simulink model "RELOrigin"  (R2022a)
settings: configuration reference "ChildModel" (kept outside this file)
libraries: simulink x4
(part 1 of 2)
settings Model: Creator=Seong Thai  LastModifiedBy=PC
settings ConfigSetRef: SourceName=ChildModel  SourceLocation=Base Workspace

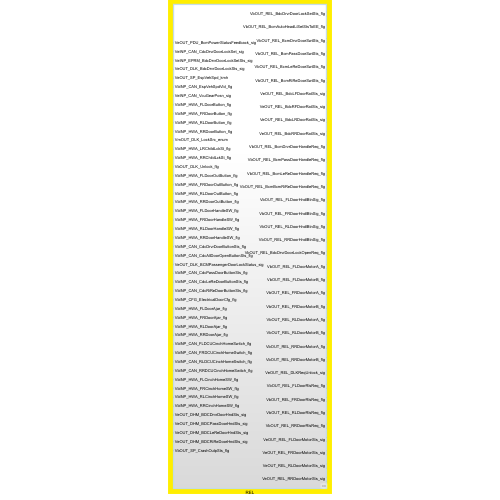
[thumbnail: Simulink's stored preview of the top-level diagram]
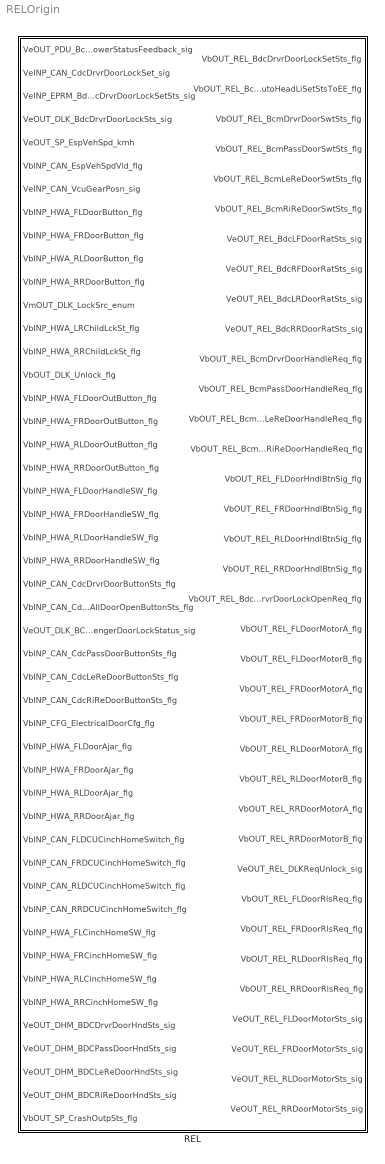
== system RELOrigin ==
  REL : Subsystem

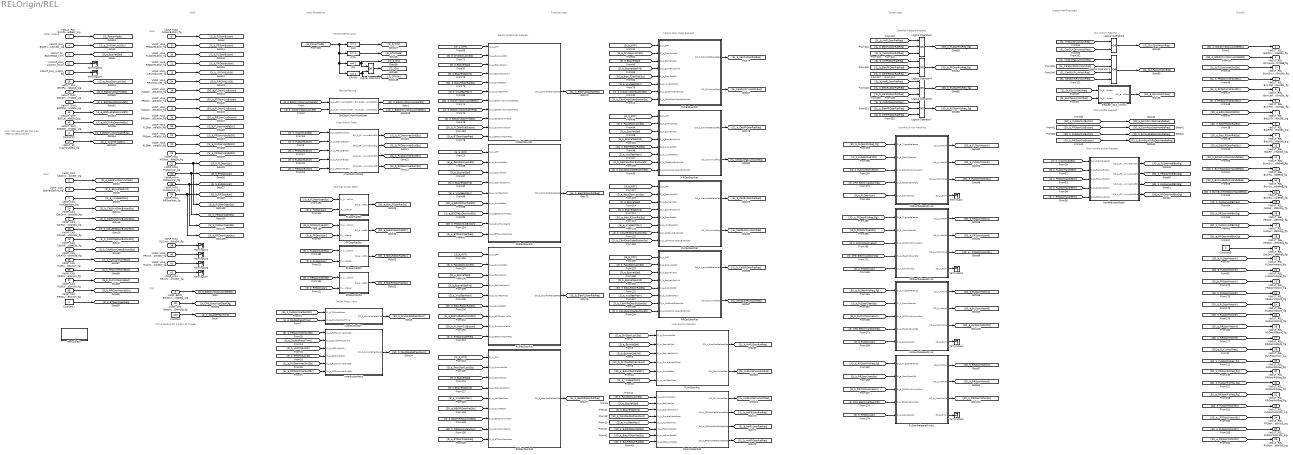
== system RELOrigin/REL ==
  note: Only NFC and BT got this Req
      | //830 no need present
  note: //Time Pending for 2 Press as Trigger
  note: CAN
  note: HWA
  note: Function Logic
  note: Input
  note: Output
  note: Input-Presetting
  note: Other Module
  note: CFG
  note: PowerMode Divation
  note: Inner Button Request
  note: Setting Passing
  note: Inner Button State
  note: Double Press Valid
  note: DoorRat Actual State
  note: Driver Logic
  note: Output Handling Logic
  note: DLK Unlock Request
  note: Door Handle Request
  note: Door Handle Button Request
  note: Electro Slide Open Request
  note: Central Door Open Request
  note: DoorRat Release Request
  note: DoorRat Driver Handling
  VeOUT_PDU_BcmPowerStatusFeedback_sig : Inport
  VeINP_CAN_CdcDrvrDoorLockSet_sig : Inport  Port=2
  VeINP_EPRM_BdcDrvrDoorLockSetSts_sig : Inport  Port=3
  VeOUT_DLK_BdcDrvrDoorLockSts_sig : Inport  Port=4
  VeOUT_SP_EspVehSpd_kmh : Inport  Port=5
  VbINP_CAN_EspVehSpdVld_flg : Inport  Port=6
  VeINP_CAN_VcuGearPosn_sig : Inport  Port=7
  VbINP_HWA_FLDoorButton_flg : Inport  Port=8
  VbINP_HWA_FRDoorButton_flg : Inport  Port=9
  VbINP_HWA_RLDoorButton_flg : Inport  Port=10
  VbINP_HWA_RRDoorButton_flg : Inport  Port=11
  VmOUT_DLK_LockSrc_enum : Inport  Port=12
  VbINP_HWA_LRChildLckSt_flg : Inport  Port=13
  VbINP_HWA_RRChildLckSt_flg : Inport  Port=14
  VbOUT_DLK_Unlock_flg : Inport  Port=15
  VbINP_HWA_FLDoorOutButton_flg : Inport  Port=16
  VbINP_HWA_FRDoorOutButton_flg : Inport  Port=17
  VbINP_HWA_RLDoorOutButton_flg : Inport  Port=18
  VbINP_HWA_RRDoorOutButton_flg : Inport  Port=19
  VbINP_HWA_FLDoorHandleSW_flg : Inport  Port=20
  VbINP_HWA_FRDoorHandleSW_flg : Inport  Port=21
  VbINP_HWA_RLDoorHandleSW_flg : Inport  Port=22
  VbINP_HWA_RRDoorHandleSW_flg : Inport  Port=23
  VbINP_CAN_CdcDrvrDoorButtonSts_flg : Inport  Port=24
  VbINP_CAN_CdcAllDoorOpenButtonSts_flg : Inport  Port=25
  VeOUT_DLK_BCMPassengerDoorLockStatus_sig : Inport  Port=26
  VbINP_CAN_CdcPassDoorButtonSts_flg : Inport  Port=27
  VbINP_CAN_CdcLeReDoorButtonSts_flg : Inport  Port=28
  VbINP_CAN_CdcRiReDoorButtonSts_flg : Inport  Port=29
  VbINP_CFG_ElectricalDoorCfg_flg : Inport  Port=30
  VbINP_HWA_FLDoorAjar_flg : Inport  Port=31
  VbINP_HWA_FRDoorAjar_flg : Inport  Port=32
  VbINP_HWA_RLDoorAjar_flg : Inport  Port=33
  VbINP_HWA_RRDoorAjar_flg : Inport  Port=34
  VbINP_CAN_FLDCUCinchHomeSwitch_flg : Inport  Port=35
  VbINP_CAN_FRDCUCinchHomeSwitch_flg : Inport  Port=36
  VbINP_CAN_RLDCUCinchHomeSwitch_flg : Inport  Port=37
  VbINP_CAN_RRDCUCinchHomeSwitch_flg : Inport  Port=38
  VbINP_HWA_FLCinchHomeSW_flg : Inport  Port=39
  VbINP_HWA_FRCinchHomeSW_flg : Inport  Port=40
  VbINP_HWA_RLCinchHomeSW_flg : Inport  Port=41
  VbINP_HWA_RRCinchHomeSW_flg : Inport  Port=42
  VeOUT_DHM_BDCDrvrDoorHndSts_sig : Inport  Port=43
  VeOUT_DHM_BDCPassDoorHndSts_sig : Inport  Port=44
  VeOUT_DHM_BDCLeReDoorHndSts_sig : Inport  Port=45
  VeOUT_DHM_BDCRiReDoorHndSts_sig : Inport  Port=46
  VbOUT_SP_CrashOutpSts_flg : Inport  Port=47
  CRANK : simulink/Logic and Bit Operations/Compare To Constant  relop===  const=3  OutDataTypeStr=boolean
  Constant : Constant  Value=200
  Constant1 : Constant  Value=0  OutDataTypeStr=uint8
  Constant2 : Constant  Value=0  OutDataTypeStr=boolean
  Constant3 : Constant  Value=0  OutDataTypeStr=boolean
  DrvDoorUnlockAutoOpen : Stateflow chart  TreatAsAtomicUnit=on
  FLCenDoorRat : Stateflow chart  TreatAsAtomicUnit=on
  FLDoorRatSts : Truth Table  TreatAsAtomicUnit=on
  FLDoorReleaseDriver : Stateflow chart  TreatAsAtomicUnit=on
  FLElecDoorRat : Stateflow chart  TreatAsAtomicUnit=on
  FLInnDoorRat : Stateflow chart  TreatAsAtomicUnit=on
  FRCenDoorRat : Stateflow chart  TreatAsAtomicUnit=on
  FRDoorRatSts : Truth Table  TreatAsAtomicUnit=on
  FRDoorReleaseDriver : Stateflow chart  TreatAsAtomicUnit=on
  FRElecDoorRat : Stateflow chart  TreatAsAtomicUnit=on
      settings: PortSchema="{\"entries\":[{\"content\":{\"sides\":[{\"content\":{\"connectorIds\":[\"In1\",\"In2\",\"In3\",\"In4\",\"In6\",\"In5\",\"In7\",\"In8\",\"In9\"]},\"type\":\"ConnectorPlacement.EquallySpacedRectSide\",\"uuid\":\"212e0ac4-578e-4dce-a8b0-108228799b81\"},{\"content\":{\"connectorIds\":[\"Out1\"],\"side\":\"RIGHT\"},\"type\":\"ConnectorPlacement.EquallySpacedRectSide\",\"uuid\":\"8fdf6a0d-489b-40c2-bb8d-375db94844e2\"},{\"content\":{\"connectorIds\":[],\"side\":\"TOP\"},\"type\":\"ConnectorPlacement.EquallySpacedRectSide\",\"uuid\":\"a80be6d9-6bfe-49a2-ae65-45f3c0c1dec5\"}]},\"type\":\"ConnectorPlacement.EquallySpacedConnector\",\"uuid\":\"25043fbd-39b7-455b-b12b-f3efbe7587dc\"}],\"packageUris\":[\"http://schema.mathworks.com/mf0/Connector/R2020b\"],\"version\":\"1.0\"}"
  HandleButtonState : Stateflow chart  TreatAsAtomicUnit=on
  InnerButtonDrv : Stateflow chart  TreatAsAtomicUnit=on
  InnerButtonPass : Stateflow chart  TreatAsAtomicUnit=on
  InnerButtonState : Stateflow chart  TreatAsAtomicUnit=on
  Logical Operator1 : Logic  Operator=OR  Inputs=4  AllPortsSameDT=off  OutDataTypeStr=boolean
  Logical Operator{2,4,6..7} (4 alike) : Logic  Operator=OR  Inputs=3  AllPortsSameDT=off  OutDataTypeStr=boolean
  Logical Operator3 : Logic  Operator=OR  AllPortsSameDT=off  OutDataTypeStr=boolean
  Logical Operator5 : Logic  Operator=OR  AllPortsSameDT=off  OutDataTypeStr=boolean
  "OFF " : simulink/Logic and Bit Operations/Compare To Constant  relop===  const=0  OutDataTypeStr=boolean
  ON : simulink/Logic and Bit Operations/Compare To Constant  relop===  const=2  OutDataTypeStr=boolean
  OTA : simulink/Logic and Bit Operations/Compare To Constant  relop===  const=1  OutDataTypeStr=boolean
  PassInnDoorRat : Stateflow chart  TreatAsAtomicUnit=on
      settings: PortSchema="{\"entries\":[{\"content\":{\"sides\":[{\"content\":{\"connectorIds\":[\"In1\",\"In2\",\"In3\",\"In4\",\"In6\",\"In5\",\"In8\",\"In7\"]},\"type\":\"ConnectorPlacement.EquallySpacedRectSide\",\"uuid\":\"5836de3c-4cf2-45a4-8dc0-e048cbbd381d\"},{\"content\":{\"connectorIds\":[\"Out1\",\"Out2\",\"Out3\",\"Out4\"],\"side\":\"RIGHT\"},\"type\":\"ConnectorPlacement.EquallySpacedRectSide\",\"uuid\":\"b6d6f1b8-f80b-4d0e-a26e-7cda05dade9a\"},{\"content\":{\"connectorIds\":[],\"side\":\"TOP\"},\"type\":\"ConnectorPlacement.EquallySpacedRectSide\",\"uuid\":\"870e6a56-16d5-491b-84d0-76547b1cbcf9\"}]},\"type\":\"ConnectorPlacement.EquallySpacedConnector\",\"uuid\":\"60f0a081-1e33-4aae-8a09-fe9fb7bd0b5c\"}],\"packageUris\":[\"http://schema.mathworks.com/mf0/Connector/R2020b\"],\"version\":\"1.0\"}"
  RLCenDoorRat : Stateflow chart  TreatAsAtomicUnit=on
  RLDoorRatSts : Truth Table  TreatAsAtomicUnit=on
  RLDoorReleaseDriver : Stateflow chart  TreatAsAtomicUnit=on
  RLDoorReleaseDriver1 : Stateflow chart  TreatAsAtomicUnit=on
  RLElecDoorRat : Stateflow chart  TreatAsAtomicUnit=on
      settings: PortSchema="{\"entries\":[{\"content\":{\"sides\":[{\"content\":{\"connectorIds\":[\"In1\",\"In2\",\"In3\",\"In4\",\"In6\",\"In5\",\"In7\",\"In8\",\"In9\"]},\"type\":\"ConnectorPlacement.EquallySpacedRectSide\",\"uuid\":\"212e0ac4-578e-4dce-a8b0-108228799b81\"},{\"content\":{\"connectorIds\":[\"Out1\"],\"side\":\"RIGHT\"},\"type\":\"ConnectorPlacement.EquallySpacedRectSide\",\"uuid\":\"8fdf6a0d-489b-40c2-bb8d-375db94844e2\"},{\"content\":{\"connectorIds\":[],\"side\":\"TOP\"},\"type\":\"ConnectorPlacement.EquallySpacedRectSide\",\"uuid\":\"a80be6d9-6bfe-49a2-ae65-45f3c0c1dec5\"}]},\"type\":\"ConnectorPlacement.EquallySpacedConnector\",\"uuid\":\"25043fbd-39b7-455b-b12b-f3efbe7587dc\"}],\"packageUris\":[\"http://schema.mathworks.com/mf0/Connector/R2020b\"],\"version\":\"1.0\"}"
  RRCenDoorRat : Stateflow chart  TreatAsAtomicUnit=on
  RRDoorRatSts : Truth Table  TreatAsAtomicUnit=on
  RRElecDoorRat : Stateflow chart  TreatAsAtomicUnit=on
      settings: PortSchema="{\"entries\":[{\"content\":{\"sides\":[{\"content\":{\"connectorIds\":[\"In1\",\"In2\",\"In3\",\"In4\",\"In6\",\"In5\",\"In7\",\"In8\",\"In9\"]},\"type\":\"ConnectorPlacement.EquallySpacedRectSide\",\"uuid\":\"212e0ac4-578e-4dce-a8b0-108228799b81\"},{\"content\":{\"connectorIds\":[\"Out1\"],\"side\":\"RIGHT\"},\"type\":\"ConnectorPlacement.EquallySpacedRectSide\",\"uuid\":\"8fdf6a0d-489b-40c2-bb8d-375db94844e2\"},{\"content\":{\"connectorIds\":[],\"side\":\"TOP\"},\"type\":\"ConnectorPlacement.EquallySpacedRectSide\",\"uuid\":\"a80be6d9-6bfe-49a2-ae65-45f3c0c1dec5\"}]},\"type\":\"ConnectorPlacement.EquallySpacedConnector\",\"uuid\":\"25043fbd-39b7-455b-b12b-f3efbe7587dc\"}],\"packageUris\":[\"http://schema.mathworks.com/mf0/Connector/R2020b\"],\"version\":\"1.0\"}"
  Recycle Bin : Subsystem
  Request_DLK_Unlock : Stateflow chart  TreatAsAtomicUnit=on
  Terminator{,1..9} (10 alike) : Terminator
  VbOUT_REL_BdcDrvrDoorLockSetSts_flg : Outport
  VbOUT_REL_BcmAutoHeadLiSetStsToEE_flg : Outport  Port=2
  VbOUT_REL_BcmDrvrDoorSwtSts_flg : Outport  Port=3
  VbOUT_REL_BcmPassDoorSwtSts_flg : Outport  Port=4
  VbOUT_REL_BcmLeReDoorSwtSts_flg : Outport  Port=5
  VbOUT_REL_BcmRiReDoorSwtSts_flg : Outport  Port=6
  VeOUT_REL_BdcLFDoorRatSts_sig : Outport  Port=7
  VeOUT_REL_BdcRFDoorRatSts_sig : Outport  Port=8
  VeOUT_REL_BdcLRDoorRatSts_sig : Outport  Port=9
  VeOUT_REL_BdcRRDoorRatSts_sig : Outport  Port=10
  VbOUT_REL_BcmDrvrDoorHandleReq_flg : Outport  Port=11
  VbOUT_REL_BcmPassDoorHandleReq_flg : Outport  Port=12
  VbOUT_REL_BcmLeReDoorHandleReq_flg : Outport  Port=13
  VbOUT_REL_BcmBcmRiReDoorHandleReq_flg : Outport  Port=14
  VbOUT_REL_FLDoorHndlBtnSig_flg : Outport  Port=15
  VbOUT_REL_FRDoorHndlBtnSig_flg : Outport  Port=16
  VbOUT_REL_RLDoorHndlBtnSig_flg : Outport  Port=17
  VbOUT_REL_RRDoorHndlBtnSig_flg : Outport  Port=18
  VbOUT_REL_BdcDrvrDoorLockOpenReq_flg : Outport  Port=19
  VbOUT_REL_FLDoorMotorA_flg : Outport  Port=20
  VbOUT_REL_FLDoorMotorB_flg : Outport  Port=21
  VbOUT_REL_FRDoorMotorA_flg : Outport  Port=22
  VbOUT_REL_FRDoorMotorB_flg : Outport  Port=23
  VbOUT_REL_RLDoorMotorA_flg : Outport  Port=24
  VbOUT_REL_RLDoorMotorB_flg : Outport  Port=25
  VbOUT_REL_RRDoorMotorA_flg : Outport  Port=26
  VbOUT_REL_RRDoorMotorB_flg : Outport  Port=27
  VeOUT_REL_DLKReqUnlock_sig : Outport  Port=28
  VbOUT_REL_FLDoorRlsReq_flg : Outport  Port=29
  VbOUT_REL_FRDoorRlsReq_flg : Outport  Port=30
  VbOUT_REL_RLDoorRlsReq_flg : Outport  Port=31
  VbOUT_REL_RRDoorRlsReq_flg : Outport  Port=32
  VeOUT_REL_FLDoorMotorSts_sig : Outport  Port=33
  VeOUT_REL_FRDoorMotorSts_sig : Outport  Port=34
  VeOUT_REL_RLDoorMotorSts_sig : Outport  Port=35
  VeOUT_REL_RRDoorMotorSts_sig : Outport  Port=36
  wires:
  "OFF "/1 -> [SI_b_OFF]
  [SI_PowerMode] -> "OFF "/1, CRANK/1, ON/1, OTA/1
  ON/1 -> [SI_b_ON], Logical Operator3/1
  CRANK/1 -> [SI_CRANK], Logical Operator3/2
  Logical Operator3/1 -> [SI_IGN]
  OTA/1 -> [SI_OTAMode]
  VeINP_EPRM_BdcDrvrDoorLockSetSts_sig/1 -> [SI_e_BdcDrvrDoorLockSetSts]
  [SO_b_BdcDrvrDoorLockSetSts] -> VbOUT_REL_BdcDrvrDoorLockSetSts_flg/1
  [SI_e_BdcDrvrDoorLockSetSts] -> DrvDoorUnlockAutoOpen/1(SI_e_BdcDrvrDoorLockSetSts)
  DrvDoorUnlockAutoOpen/1(SO_b_BdcDrvrDoorLockSetSts) -> [SO_b_BdcDrvrDoorLockSetSts]
  VeINP_CAN_CdcDrvrDoorLockSet_sig/1 -> [SI_e_CdcDrvrDoorLockSet]
  [SI_e_CdcDrvrDoorLockSet] -> DrvDoorUnlockAutoOpen/2(SI_e_CdcDrvrDoorLockSet)
  VeOUT_DLK_BdcDrvrDoorLockSts_sig/1 -> [SI_e_DrvDoorLockSts]
  VeOUT_SP_EspVehSpd_kmh/1 -> [SI_e_EspVehSpd]
  VbINP_CAN_EspVehSpdVld_flg/1 -> [SI_b_EspVehSpdVld]
  VbINP_HWA_FLDoorButton_flg/1 -> [SI_b_FLDoorButton]
  [SI_e_DoublePressTime] -> InnerButtonDrv/2(SI_e_DoublePressTime)
  Constant/1 -> [SI_e_DoublePressTime]
  InnerButtonDrv/1(SO_b_DoublePressSucc) -> [SO_b_DrvDoublePressSucc]
  [SI_e_EspVehSpd] -> FLInnDoorRat/2(SI_e_EspVehSpd)
  [SI_b_EspVehSpdVld] -> FLInnDoorRat/3(SI_b_EspVehSpdVld)
  [SO_b_DrvDoublePressSucc] -> FLInnDoorRat/4(SI_b_DoublePressSucc)
  VeINP_CAN_VcuGearPosn_sig/1 -> [SI_e_VcuGearPosn]
  [SI_e_VcuGearPosn] -> FLInnDoorRat/6(SI_e_VcuGearPosn)
  VeOUT_DLK_BCMPassengerDoorLockStatus_sig/1 -> [SI_e_PassDoorLockSts]
  [SI_e_DrvDoorLockSts] -> FLInnDoorRat/1(SI_e_DoorLockSts)
  [SI_e_EspVehSpd] -> PassInnDoorRat/2(SI_e_EspVehSpd)
  [SI_b_EspVehSpdVld] -> PassInnDoorRat/3(SI_b_EspVehSpdVld)
  [SI_e_PassDoorLockSts] -> PassInnDoorRat/1(SI_e_DoorLockSts)
  [SI_e_VcuGearPosn] -> PassInnDoorRat/6(SI_e_VcuGearPosn)
  [SI_e_DoublePressTime] -> InnerButtonPass/2(SI_e_DoublePressTime)
  VbINP_HWA_FRDoorButton_flg/1 -> [SI_b_FRDoorButton]
  VbINP_HWA_LRChildLckSt_flg/1 -> [SI_b_LRChildLckSt]
  VbINP_HWA_RRChildLckSt_flg/1 -> [SI_b_RRChildLckSt]
  [SI_b_LRChildLckSt] -> InnerButtonPass/3(SI_b_LRChildLckSt)
  [SI_b_RRChildLckSt] -> InnerButtonPass/4(SI_b_RRChildLckSt)
  VbINP_CAN_CdcDrvrDoorButtonSts_flg/1 -> [SI_b_CdcDrvrDoorButtonSts]
  VbINP_CAN_CdcPassDoorButtonSts_flg/1 -> [SI_b_CdcPassDoorButtonSts]
  VbINP_CAN_CdcLeReDoorButtonSts_flg/1 -> [SI_b_CdcLeReDoorButtonSts]
  VbINP_CAN_CdcRiReDoorButtonSts_flg/1 -> [SI_b_CdcRiReDoorButtonSts]
  VbINP_HWA_RLDoorButton_flg/1 -> [SI_b_RLDoorButton]
  VbINP_HWA_RRDoorButton_flg/1 -> [SI_b_RRDoorButton]
  [SL_b_FLDoorInnerSwtSts] -> InnerButtonDrv/1(SI_b_FLDoorButton)
  [SL_b_FRDoorInnerSwtSts] -> InnerButtonPass/1(SL_b_FRDoorInnerSwtSts)
  [SL_b_RLDoorInnerSwtSts] -> InnerButtonPass/5(SL_b_RLDoorInnerSwtSts)
  [SL_b_RRDoorInnerSwtSts] -> InnerButtonPass/6(SL_b_RRDoorInnerSwtSts)
  InnerButtonPass/1(SO_b_DoublePressSucc) -> [SO_b_PassDoublePressSucc]
  [SO_b_PassDoublePressSucc] -> PassInnDoorRat/4(SI_b_DoublePressSucc)
  VbINP_HWA_FLDoorAjar_flg/1 -> [SI_b_FLDoorOpenSts], [SI_b_FLDoorAjar]
  VbINP_HWA_FRDoorAjar_flg/1 -> [SI_b_FRDoorOpenSts], [SI_b_FRDoorAjar]
  VbINP_HWA_RLDoorAjar_flg/1 -> [SI_b_RLDoorOpenSts], [SI_b_RLDoorAjar]
  VbINP_HWA_RRDoorAjar_flg/1 -> [SI_b_RRDoorOpenSts], [SI_b_RRDoorAjar]
  [SI_b_FLDoorOpenSts] -> FLDoorRatSts/1(SI_b_DoorAjarSwt)
  [SI_b_RRDoorAjar] -> RRDoorRatSts/2(SI_b_DoorSlideAjar)
  [SI_b_RLDoorAjar] -> RLDoorRatSts/2(SI_b_DoorSlideAjar)
  [SI_b_FRDoorAjar] -> FRDoorRatSts/2(SI_b_DoorSlideAjar)
  [SI_b_FLDoorAjar] -> FLDoorRatSts/2(SI_b_DoorSlideAjar)
  [SI_b_FRDoorOpenSts] -> FRDoorRatSts/1(SI_b_DoorAjarSwt)
  [SI_b_RLDoorOpenSts] -> RLDoorRatSts/1(SI_b_DoorAjarSwt)
  [SI_b_RRDoorOpenSts] -> RRDoorRatSts/1(SI_b_DoorAjarSwt)
  [SO_e_BdcLFDoorRatSts] -> VeOUT_REL_BdcLFDoorRatSts_sig/1
  [SO_e_BdcRFDoorRatSts] -> VeOUT_REL_BdcRFDoorRatSts_sig/1
  [SO_e_BdcLRDoorRatSts] -> VeOUT_REL_BdcLRDoorRatSts_sig/1
  [SO_e_BdcRRDoorRatSts] -> VeOUT_REL_BdcRRDoorRatSts_sig/1
  FLDoorRatSts/1(SO_e_DoorRatSts) -> [SO_e_BdcLFDoorRatSts]
  FRDoorRatSts/1(SO_e_DoorRatSts) -> [SO_e_BdcRFDoorRatSts]
  RRDoorRatSts/1(SO_e_DoorRatSts) -> [SO_e_BdcRRDoorRatSts]
  RLDoorRatSts/1(SO_e_DoorRatSts) -> [SO_e_BdcLRDoorRatSts]
  [SO_e_BdcLFDoorRatSts] -> FLInnDoorRat/5(SI_e_DoorRatSts)
  [SO_e_BdcRFDoorRatSts] -> PassInnDoorRat/5(SI_e_FRDoorRatSts)
  [SO_e_BdcLRDoorRatSts] -> PassInnDoorRat/8(SI_e_RLDoorRatSts)
  [SO_e_BdcRRDoorRatSts] -> PassInnDoorRat/7(SI_e_RRDoorRatSts)
  [SL_b_FLDoorInnerSwtSts] -> VbOUT_REL_BcmDrvrDoorSwtSts_flg/1
  [SL_b_FRDoorInnerSwtSts] -> VbOUT_REL_BcmPassDoorSwtSts_flg/1
  [SL_b_RLDoorInnerSwtSts] -> VbOUT_REL_BcmLeReDoorSwtSts_flg/1
  [SL_b_RRDoorInnerSwtSts] -> VbOUT_REL_BcmRiReDoorSwtSts_flg/1
  FLInnDoorRat/2(SO_DLKUnlockReq) -> [SL_InnDLKDrvUnlockReq]
  PassInnDoorRat/1(SO_DLKUnlockReq) -> [SL_InnDLKPassUnlockReq]
  [SL_DLKDrvUnlockReq] -> Request_DLK_Unlock/1(SL_DLKDrvUnlockReq)
  [SL_DLKPassUnlockReq] -> Request_DLK_Unlock/2(SL_DLKPassUnlockReq)
  Request_DLK_Unlock/1(SO_e_DLKUnlockReq) -> [SO_e_DLKUnlockReq]
  [SO_e_DLKUnlockReq] -> VeOUT_REL_DLKReqUnlock_sig/1
  VbINP_HWA_FLDoorHandleSW_flg/1 -> [SI_b_FLDoorHandleSW]
  VbINP_HWA_FRDoorHandleSW_flg/1 -> [SI_b_FRDoorHandleSW]
  VbINP_HWA_RLDoorHandleSW_flg/1 -> [SI_b_RLDoorHandleSW]
  VbINP_HWA_RRDoorHandleSW_flg/1 -> [SI_b_RRDoorHandleSW]
  [SO_b_BcmDrvrDoorHandleReq] -> VbOUT_REL_BcmDrvrDoorHandleReq_flg/1
  [SO_b_BcmPassDoorHandleReq] -> VbOUT_REL_BcmPassDoorHandleReq_flg/1
  [SO_b_BcmLeReDoorHandleReq] -> VbOUT_REL_BcmLeReDoorHandleReq_flg/1
  [SO_b_BcmBcmRiReDoorHandleReq] -> VbOUT_REL_BcmBcmRiReDoorHandleReq_flg/1
  VbINP_HWA_FLDoorOutButton_flg/1 -> [SO_b_FLDoorOutButton]
  VbINP_HWA_FRDoorOutButton_flg/1 -> [SO_b_FRDoorOutButton]
  VbINP_HWA_RLDoorOutButton_flg/1 -> [SO_b_RLDoorOutButton]
  VbINP_HWA_RRDoorOutButton_flg/1 -> [SO_b_RRDoorOutButton]
  [SO_b_FLDoorHndlBtnSig] -> VbOUT_REL_FLDoorHndlBtnSig_flg/1
  [SO_b_FRDoorHndlBtnSig] -> VbOUT_REL_FRDoorHndlBtnSig_flg/1
  [SO_b_RLDoorHndlBtnSig] -> VbOUT_REL_RLDoorHndlBtnSig_flg/1
  [SO_b_RRDoorHndlBtnSig] -> VbOUT_REL_RRDoorHndlBtnSig_flg/1
  VeOUT_PDU_BcmPowerStatusFeedback_sig/1 -> [SI_PowerMode]
  [SI_e_DrvDoorLockSts] -> FLElecDoorRat/2(SI_e_DoorLockSts)
  [SI_e_EspVehSpd] -> FLElecDoorRat/3(SI_e_EspVehSpd)
  [SI_b_EspVehSpdVld] -> FLElecDoorRat/4(SI_b_EspVehSpdVld)
  [SO_e_BdcLFDoorRatSts] -> FLElecDoorRat/5(SI_e_DoorRatSts)
  [SI_e_VcuGearPosn] -> FLElecDoorRat/6(SI_e_VcuGearPosn)
  [SI_b_OFF] -> FLElecDoorRat/1(SI_b_OFF)
  [SO_b_BdcDrvrDoorLockSetSts] -> FLElecDoorRat/7(SI_b_BdcDrvrDoorLockSetSts)
  Constant2/1 -> [SI_b_BDCDrvrDoorOpenReq]
  [SI_b_BDCDrvrDoorOpenReq] -> FLElecDoorRat/8(SI_b_BDCDrvrDoorOpenReq)
  VeOUT_DHM_BDCDrvrDoorHndSts_sig/1 -> [SI_e_BDCDrvDoorHndSts]
  [SI_e_BDCDrvDoorHndSts] -> FLElecDoorRat/9(SI_e_BDCDoorHndSts)
  [SO_b_FLDoorOutButton] -> FLElecDoorRat/10(SI_b_DoorHandleSW)
  [SI_e_BTDoorOpenReq] -> FLElecDoorRat/11(SI_e_BTDoorOpenReq)
  Constant1/1 -> [SI_e_BTDoorOpenReq]
  FLCenDoorRat/2(SO_DLKUnlockReq) -> [SL_CenDLKDrvUnlockReq]
  [SO_e_BdcLFDoorRatSts] -> FLCenDoorRat/5(SI_e_DoorRatSts)
  [SI_e_DrvDoorLockSts] -> FLCenDoorRat/2(SI_e_DoorLockSts)
  [SI_e_VcuGearPosn] -> FLCenDoorRat/6(SI_e_VcuGearPosn)
  [SI_b_EspVehSpdVld] -> FLCenDoorRat/4(SI_b_EspVehSpdVld)
  [SI_e_EspVehSpd] -> FLCenDoorRat/3(SI_e_EspVehSpd)
  Logical Operator5/1 -> [SL_DLKDrvUnlockReq]
  [SL_InnDLKDrvUnlockReq] -> Logical Operator5/1
  [SL_CenDLKDrvUnlockReq] -> Logical Operator5/2
  VbINP_CAN_CdcAllDoorOpenButtonSts_flg/1 -> [SI_b_Cdc4DoorOpenButtonSts]
  [SI_b_CdcDrvrDoorButtonSts] -> FLCenDoorRat/7(SI_b_CdcDoorButtonSts)
  [SI_b_Cdc4DoorOpenButtonSts] -> FLCenDoorRat/8(SI_b_Cdc4DoorOpenButtonSts)
  [SI_b_OFF] -> FLCenDoorRat/1(SI_b_OFF)
  [SI_b_OFF] -> FRElecDoorRat/1(SI_b_OFF)
  [SI_e_VcuGearPosn] -> FRElecDoorRat/6(SI_e_VcuGearPosn)
  [SI_b_EspVehSpdVld] -> FRElecDoorRat/4(SI_b_EspVehSpdVld)
  [SI_e_EspVehSpd] -> FRElecDoorRat/3(SI_e_EspVehSpd)
  [SI_e_PassDoorLockSts] -> FRElecDoorRat/2(SI_e_DoorLockSts)
  [SO_e_BdcRFDoorRatSts] -> FRElecDoorRat/5(SI_e_DoorRatSts)
  [SI_e_BTDoorOpenReq] -> FRElecDoorRat/9(SI_e_BTDoorOpenReq)
  [SO_b_FRDoorOutButton] -> FRElecDoorRat/8(SI_b_DoorHandleSW)
  VeOUT_DHM_BDCPassDoorHndSts_sig/1 -> [SI_e_BDCPassDoorHndSts]
  [SI_e_BDCPassDoorHndSts] -> FRElecDoorRat/7(SI_e_BDCDoorHndSts)
  [SI_b_OFF] -> FRCenDoorRat/1(SI_b_OFF)
  [SI_b_Cdc4DoorOpenButtonSts] -> FRCenDoorRat/8(SI_b_Cdc4DoorOpenButtonSts)
  [SI_b_CdcPassDoorButtonSts] -> FRCenDoorRat/7(SI_b_CdcDoorButtonSts)
  [SI_e_EspVehSpd] -> FRCenDoorRat/3(SI_e_EspVehSpd)
  [SI_b_EspVehSpdVld] -> FRCenDoorRat/4(SI_b_EspVehSpdVld)
  [SI_e_VcuGearPosn] -> FRCenDoorRat/6(SI_e_VcuGearPosn)
  [SO_e_BdcRFDoorRatSts] -> FRCenDoorRat/5(SI_e_DoorRatSts)
  FRCenDoorRat/2(SO_DLKUnlockReq) -> [SL_CenDLKPassUnlockReq]
  Logical Operator1/1 -> [SL_DLKPassUnlockReq]
  [SL_InnDLKPassUnlockReq] -> Logical Operator1/1
  [SL_CenDLKPassUnlockReq] -> Logical Operator1/2
  [SI_e_PassDoorLockSts] -> FRCenDoorRat/2(SI_e_DoorLockSts)
  [SI_e_BDCLeReDoorHndSts] -> RLElecDoorRat/7(SI_e_BDCDoorHndSts)
  [SO_b_RLDoorOutButton] -> RLElecDoorRat/8(SI_b_DoorHandleSW)
  [SI_e_BTDoorOpenReq] -> RLElecDoorRat/9(SI_e_BTDoorOpenReq)
  [SO_e_BdcLRDoorRatSts] -> RLElecDoorRat/5(SI_e_DoorRatSts)
  [SI_e_PassDoorLockSts] -> RLElecDoorRat/2(SI_e_DoorLockSts)
  [SI_e_EspVehSpd] -> RLElecDoorRat/3(SI_e_EspVehSpd)
  [SI_b_EspVehSpdVld] -> RLElecDoorRat/4(SI_b_EspVehSpdVld)
  [SI_e_VcuGearPosn] -> RLElecDoorRat/6(SI_e_VcuGearPosn)
  [SI_b_OFF] -> RLElecDoorRat/1(SI_b_OFF)
  VeOUT_DHM_BDCLeReDoorHndSts_sig/1 -> [SI_e_BDCLeReDoorHndSts]
  [SI_e_PassDoorLockSts] -> RLCenDoorRat/2(SI_e_DoorLockSts)
  RLCenDoorRat/2(SO_DLKUnlockReq) -> [SL_CenDLKRLUnlockReq]
  [SO_e_BdcLRDoorRatSts] -> RLCenDoorRat/5(SI_e_DoorRatSts)
  [SI_e_VcuGearPosn] -> RLCenDoorRat/6(SI_e_VcuGearPosn)
  [SI_b_EspVehSpdVld] -> RLCenDoorRat/4(SI_b_EspVehSpdVld)
  [SI_e_EspVehSpd] -> RLCenDoorRat/3(SI_e_EspVehSpd)
  [SI_b_CdcLeReDoorButtonSts] -> RLCenDoorRat/7(SI_b_CdcDoorButtonSts)
  [SI_b_Cdc4DoorOpenButtonSts] -> RLCenDoorRat/8(SI_b_Cdc4DoorOpenButtonSts)
  [SI_b_OFF] -> RLCenDoorRat/1(SI_b_OFF)
  [SL_CenDLKRLUnlockReq] -> Logical Operator1/3
  [SI_b_OFF] -> RRElecDoorRat/1(SI_b_OFF)
  [SI_e_VcuGearPosn] -> RRElecDoorRat/6(SI_e_VcuGearPosn)
  [SI_b_EspVehSpdVld] -> RRElecDoorRat/4(SI_b_EspVehSpdVld)
  [SI_e_EspVehSpd] -> RRElecDoorRat/3(SI_e_EspVehSpd)
  [SI_e_PassDoorLockSts] -> RRElecDoorRat/2(SI_e_DoorLockSts)
  [SI_e_BTDoorOpenReq] -> RRElecDoorRat/9(SI_e_BTDoorOpenReq)
  [SO_e_BdcRRDoorRatSts] -> RRElecDoorRat/5(SI_e_DoorRatSts)
  VeOUT_DHM_BDCRiReDoorHndSts_sig/1 -> [SI_e_BDCRiReDoorHndSts]
  [SI_e_BDCRiReDoorHndSts] -> RRElecDoorRat/7(SI_e_BDCDoorHndSts)
  [SO_b_RRDoorOutButton] -> RRElecDoorRat/8(SI_b_DoorHandleSW)
  [SI_b_OFF] -> RRCenDoorRat/1(SI_b_OFF)
  [SI_b_Cdc4DoorOpenButtonSts] -> RRCenDoorRat/8(SI_b_Cdc4DoorOpenButtonSts)
  [SI_e_EspVehSpd] -> RRCenDoorRat/3(SI_e_EspVehSpd)
  [SI_b_EspVehSpdVld] -> RRCenDoorRat/4(SI_b_EspVehSpdVld)
  [SI_e_VcuGearPosn] -> RRCenDoorRat/6(SI_e_VcuGearPosn)
  [SO_e_BdcLRDoorRatSts] -> RRCenDoorRat/5(SI_e_DoorRatSts)
  RRCenDoorRat/2(SO_DLKUnlockReq) -> [SL_CenDLKRRUnlockReq]
  [SI_e_PassDoorLockSts] -> RRCenDoorRat/2(SI_e_DoorLockSts)
  [SI_b_CdcRiReDoorButtonSts] -> RRCenDoorRat/7(SI_b_CdcDoorButtonSts)
  FLInnDoorRat/1(SO_b_DoorRatRelaseReq) -> [SL_b_InnFLDoorRatReq]
  PassInnDoorRat/2(SO_b_FRDoorRatReleaseReq) -> [SL_b_InnFRDoorRatReq]
  PassInnDoorRat/3(SO_b_RLDoorRatReleaseReq) -> [SL_b_InnRLDoorRatReq]
  PassInnDoorRat/4(SO_b_RRDoorRatReleaseReq) -> [SL_b_InnRRDoorRatReq]
  FLElecDoorRat/1(SO_b_DoorRatRelaseReq) -> [SL_b_ElecFLDoorRatReq]
  FLCenDoorRat/1(SO_b_DoorRatRelaseReq) -> [SL_b_CenFLDoorRatReq]
  FRElecDoorRat/1(SO_b_DoorRatRelaseReq) -> [SL_b_ElecFRDoorRatReq]
  RLElecDoorRat/1(SO_b_DoorRatRelaseReq) -> [SL_b_ElecRLDoorRatReq]
  RRElecDoorRat/1(SO_b_DoorRatRelaseReq) -> [SL_b_ElecRRDoorRatReq]
  FRCenDoorRat/1(SO_b_DoorRatRelaseReq) -> [SL_b_CenFRDoorRatReq]
  RLCenDoorRat/1(SO_b_DoorRatRelaseReq) -> [SL_b_CenRLDoorRatReq]
  RRCenDoorRat/1(SO_b_DoorRatRelaseReq) -> [SL_b_CenRRDoorRatReq]
  [SL_CenDLKRRUnlockReq] -> Logical Operator1/4
  [SO_b_FLDoorOutButton] -> [SO_b_BcmDrvrDoorHandleReq]
  [SO_b_FRDoorOutButton] -> [SO_b_BcmPassDoorHandleReq]
  [SO_b_RLDoorOutButton] -> [SO_b_BcmLeReDoorHandleReq]
  [SO_b_RRDoorOutButton] -> [SO_b_BcmBcmRiReDoorHandleReq]
  Constant3/1 -> VbOUT_REL_BdcDrvrDoorLockOpenReq_flg/1
  [SO_b_FLDoorMotorA] -> VbOUT_REL_FLDoorMotorA_flg/1
  [SO_b_FLDoorMotorB] -> VbOUT_REL_FLDoorMotorB_flg/1
  FLDoorReleaseDriver/2(SO_b_MotorB) -> [SO_b_FLDoorMotorB]
  FLDoorReleaseDriver/1(SO_b_MotorA) -> [SO_b_FLDoorMotorA]
  [SL_b_ElecFLDoorRatReq] -> Logical Operator2/2
  [SL_b_InnFLDoorRatReq] -> Logical Operator2/1
  [SL_b_CenFLDoorRatReq] -> Logical Operator2/3
  [SL_b_InnFRDoorRatReq] -> Logical Operator4/1
  [SL_b_ElecFRDoorRatReq] -> Logical Operator4/2
  [SL_b_CenFRDoorRatReq] -> Logical Operator4/3
  [SL_b_ElecRLDoorRatReq] -> Logical Operator6/2
  [SL_b_InnRLDoorRatReq] -> Logical Operator6/1
  [SL_b_CenRLDoorRatReq] -> Logical Operator6/3
  [SL_b_InnRRDoorRatReq] -> Logical Operator7/1
  [SL_b_ElecRRDoorRatReq] -> Logical Operator7/2
  [SL_b_CenRRDoorRatReq] -> Logical Operator7/3
  [SO_b_FLDoorRlsReq_flg] -> VbOUT_REL_FLDoorRlsReq_flg/1
  [SO_b_FRDoorRlsReq_flg] -> VbOUT_REL_FRDoorRlsReq_flg/1
  [SO_b_RLDoorRlsReq_flg] -> VbOUT_REL_RLDoorRlsReq_flg/1
  [SO_b_RRDoorRlsReq_flg] -> VbOUT_REL_RRDoorRlsReq_flg/1
  Logical Operator2/1 -> [SO_b_FLDoorRlsReq_flg]
  Logical Operator7/1 -> [SO_b_RRDoorRlsReq_flg]
  Logical Operator6/1 -> [SO_b_RLDoorRlsReq_flg]
  Logical Operator4/1 -> [SO_b_FRDoorRlsReq_flg]
  [SO_b_FLDoorRlsReq_flg] -> FLDoorReleaseDriver/1(SI_b_TriggerRelease)
  [SI_b_FLDoorAjar] -> FLDoorReleaseDriver/5(SI_b_DoorAjarSts)
  VbINP_CAN_FLDCUCinchHomeSwitch_flg/1 -> [SI_b_FLCinchHomeSwt]
  VbINP_CAN_FRDCUCinchHomeSwitch_flg/1 -> [SI_b_FRCinchHomeSwt]
  VbINP_CAN_RLDCUCinchHomeSwitch_flg/1 -> [SI_b_RLCinchHomeSwt]
  VbINP_CAN_RRDCUCinchHomeSwitch_flg/1 -> [SI_b_RRCinchHomeSwt]
  [SO_b_FRDoorRlsReq_flg] -> FRDoorReleaseDriver/1(SI_b_TriggerRelease)
  [SO_b_RLDoorRlsReq_flg] -> RLDoorReleaseDriver/1(SI_b_TriggerRelease)
  [SO_b_RRDoorRlsReq_flg] -> RLDoorReleaseDriver1/1(SI_b_TriggerRelease)
  [SI_b_FRDoorAjar] -> FRDoorReleaseDriver/5(SI_b_DoorAjarSts)
  [SI_b_RRDoorAjar] -> RLDoorReleaseDriver1/5(SI_b_DoorAjarSts)
  [SI_b_FLCinchHomeSwt] -> FLDoorReleaseDriver/3(SI_b_DCUCinchHomeSwt)
  [SI_b_FRCinchHomeSwt] -> FRDoorReleaseDriver/3(SI_b_DCUCinchHomeSwt)
  [SI_b_RLCinchHomeSwt] -> RLDoorReleaseDriver/3(SI_b_DCUCinchHomeSwt)
  [SI_b_RRCinchHomeSwt] -> RLDoorReleaseDriver1/3(SI_b_DCUCinchHomeSwt)
  VbINP_CFG_ElectricalDoorCfg_flg/1 -> [SI_CFG_ElectricalDoorCfg]
  [SI_CFG_ElectricalDoorCfg] -> FLDoorReleaseDriver/4(SI_b_ElectricDoorCfg)
  [SI_CFG_ElectricalDoorCfg] -> FRDoorReleaseDriver/4(SI_b_ElectricDoorCfg)
  [SI_CFG_ElectricalDoorCfg] -> RLDoorReleaseDriver/4(SI_b_ElectricDoorCfg)
  [SI_CFG_ElectricalDoorCfg] -> RLDoorReleaseDriver1/4(SI_b_ElectricDoorCfg)
  [SO_b_FRDoorMotorB] -> VbOUT_REL_FRDoorMotorB_flg/1
  [SO_b_RLDoorMotorB] -> VbOUT_REL_RLDoorMotorB_flg/1
  [SO_b_RRDoorMotorB] -> VbOUT_REL_RRDoorMotorB_flg/1
  [SO_b_FRDoorMotorA] -> VbOUT_REL_FRDoorMotorA_flg/1
  [SO_b_RLDoorMotorA] -> VbOUT_REL_RLDoorMotorA_flg/1
  [SO_b_RRDoorMotorA] -> VbOUT_REL_RRDoorMotorA_flg/1
  RLDoorReleaseDriver1/1(SO_b_MotorA) -> [SO_b_RRDoorMotorA]
  RLDoorReleaseDriver1/2(SO_b_MotorB) -> [SO_b_RRDoorMotorB]
  RLDoorReleaseDriver/2(SO_b_MotorB) -> [SO_b_RLDoorMotorB]
  RLDoorReleaseDriver/1(SO_b_MotorA) -> [SO_b_RLDoorMotorA]
  FRDoorReleaseDriver/1(SO_b_MotorA) -> [SO_b_FRDoorMotorA]
  FRDoorReleaseDriver/2(SO_b_MotorB) -> [SO_b_FRDoorMotorB]
  [SO_e_FLDoorMotorSts] -> VeOUT_REL_FLDoorMotorSts_sig/1
  [SO_e__FRDoorMotorSts] -> VeOUT_REL_FRDoorMotorSts_sig/1
  [SO_e_RLDoorMotorSts] -> VeOUT_REL_RLDoorMotorSts_sig/1
  [SO_e_RRDoorMotorSts] -> VeOUT_REL_RRDoorMotorSts_sig/1
  FLDoorReleaseDriver/3(SO_e_MotorMode) -> [SO_e_FLDoorMotorSts]
  FRDoorReleaseDriver/3(SO_e_MotorMode) -> [SO_e__FRDoorMotorSts]
  RLDoorReleaseDriver/3(SO_e_MotorMode) -> [SO_e_RLDoorMotorSts]
  RLDoorReleaseDriver1/3(SO_e_MotorMode) -> [SO_e_RRDoorMotorSts]
  FLDoorReleaseDriver/4(SO_b_Error) -> Terminator/1
  FRDoorReleaseDriver/4(SO_b_Error) -> Terminator1/1
  RLDoorReleaseDriver/4(SO_b_Error) -> Terminator2/1
  RLDoorReleaseDriver1/4(SO_b_Error) -> Terminator3/1
  VbINP_HWA_FLCinchHomeSW_flg/1 -> Terminator4/1
  VbINP_HWA_FRCinchHomeSW_flg/1 -> Terminator5/1
  VbINP_HWA_RLCinchHomeSW_flg/1 -> Terminator6/1
  VbINP_HWA_RRCinchHomeSW_flg/1 -> Terminator7/1
  VmOUT_DLK_LockSrc_enum/1 -> Terminator8/1
  VbOUT_DLK_Unlock_flg/1 -> Terminator9/1
  VbOUT_SP_CrashOutpSts_flg/1 -> [SI_b_CrashOutpSts]
  [SI_b_FLDoorOpenSts] -> FLDoorReleaseDriver/2(SI_b_DoorOpenSts)
  [SI_b_FRDoorOpenSts] -> FRDoorReleaseDriver/2(SI_b_DoorOpenSts)
  [SI_b_RLDoorOpenSts] -> RLDoorReleaseDriver/2(SI_b_DoorOpenSts)
  [SI_b_RLDoorAjar] -> RLDoorReleaseDriver/5(SI_b_DoorAjarSts)
  [SI_b_RRDoorOpenSts] -> RLDoorReleaseDriver1/2(SI_b_DoorOpenSts)
  [SI_b_CrashOutpSts] -> InnerButtonState/1(SI_b_CrashOutpSts)
  [SI_b_FLDoorButton] -> InnerButtonState/2(SI_b_FLDoorButton)
  [SI_b_FRDoorButton] -> InnerButtonState/3(SI_b_FRDoorButton)
  [SI_b_RLDoorButton] -> InnerButtonState/4(SI_b_RLDoorButton)
  [SI_b_RRDoorButton] -> InnerButtonState/5(SI_b_RRDoorButton)
  InnerButtonState/1(SO_b_FLDoorInnerSwtSts) -> [SL_b_FLDoorInnerSwtSts]
  InnerButtonState/2(SO_b_FRDoorInnerSwtSts) -> [SL_b_FRDoorInnerSwtSts]
  InnerButtonState/3(SO_b_RLDoorInnerSwtSts) -> [SL_b_RLDoorInnerSwtSts]
  InnerButtonState/4(SO_b_RRDoorInnerSwtSts) -> [SL_b_RRDoorInnerSwtSts]
  [SI_b_CrashOutpSts] -> HandleButtonState/1(SI_b_CrashOutpSts)
  [SI_b_RRDoorHandleSW] -> HandleButtonState/5(SI_b_RRDoorButton)
  [SI_b_RLDoorHandleSW] -> HandleButtonState/4(SI_b_RLDoorButton)
  [SI_b_FRDoorHandleSW] -> HandleButtonState/3(SI_b_FRDoorButton)
  [SI_b_FLDoorHandleSW] -> HandleButtonState/2(SI_b_FLDoorButton)
  HandleButtonState/3(SO_b_RLDoorInnerSwtSts) -> [SO_b_RLDoorHndlBtnSig]
  HandleButtonState/2(SO_b_FRDoorInnerSwtSts) -> [SO_b_FRDoorHndlBtnSig]
  HandleButtonState/4(SO_b_RRDoorInnerSwtSts) -> [SO_b_RRDoorHndlBtnSig]
  HandleButtonState/1(SO_b_FLDoorInnerSwtSts) -> [SO_b_FLDoorHndlBtnSig]
  DrvDoorUnlockAutoOpen/2(SO_b_E2BdcDrvrDoorLockSetSts) -> [SO_b_E2BdcDrvrDoorLockSetSts]
  [SO_b_E2BdcDrvrDoorLockSetSts] -> VbOUT_REL_BcmAutoHeadLiSetStsToEE_flg/1

== system RELOrigin/REL/Recycle Bin ==

== stateflow chart RELOrigin/REL/InnerButtonState ==
  state Initial
    en:
    SO_b_FLDoorInnerSwtSts=SI_b_FLDoorButton;
    SO_b_FRDoorInnerSwtSts=SI_b_FRDoorButton;
    SO_b_RLDoorInnerSwtSts=SI_b_RLDoorButton;
    SO_b_RRDoorInnerSwtSts=SI_b_RRDoorButton;
    du:
    SO_b_FLDoorInnerSwtSts=SI_b_FLDoorButton;
    SO_b_FRDoorInnerSwtSts=SI_b_FRDoorButton;
    SO_b_RLDoorInnerSwtSts=SI_b_RLDoorButton;
    SO_b_RRDoorInnerSwtSts=SI_b_RRDoorButton;
  state ONCE
    en:
    SO_b_FLDoorInnerSwtSts=0;
    SO_b_FRDoorInnerSwtSts=0;
    SO_b_RLDoorInnerSwtSts=0;
    SO_b_RRDoorInnerSwtSts=0;
  (default) -> Initial
  Initial -> ONCE : [hasChangedTo(SI_b_CrashOutpSts,1)]
  ONCE -> Initial : [after(10000,tick)]
  data: SO_b_FLDoorInnerSwtSts output boolean; SI_b_CrashOutpSts input boolean; SI_b_FLDoorButton input boolean; SI_b_FRDoorButton input boolean; SI_b_RLDoorButton input boolean; SI_b_RRDoorButton input boolean; SO_b_FRDoorInnerSwtSts output boolean; SO_b_RLDoorInnerSwtSts output boolean; SO_b_RRDoorInnerSwtSts output boolean

== stateflow chart RELOrigin/REL/HandleButtonState ==
  state Initial
    en:
    SO_b_FLDoorInnerSwtSts=SI_b_FLDoorButton;
    SO_b_FRDoorInnerSwtSts=SI_b_FRDoorButton;
    SO_b_RLDoorInnerSwtSts=SI_b_RLDoorButton;
    SO_b_RRDoorInnerSwtSts=SI_b_RRDoorButton;
    du:
    SO_b_FLDoorInnerSwtSts=SI_b_FLDoorButton;
    SO_b_FRDoorInnerSwtSts=SI_b_FRDoorButton;
    SO_b_RLDoorInnerSwtSts=SI_b_RLDoorButton;
    SO_b_RRDoorInnerSwtSts=SI_b_RRDoorButton;
  state ONCE
    en:
    SO_b_FLDoorInnerSwtSts=0;
    SO_b_FRDoorInnerSwtSts=0;
    SO_b_RLDoorInnerSwtSts=0;
    SO_b_RRDoorInnerSwtSts=0;
  (default) -> Initial
  Initial -> ONCE : [hasChangedTo(SI_b_CrashOutpSts,1)]
  ONCE -> Initial : [after(10000,tick)]
  data: SO_b_FLDoorInnerSwtSts output boolean; SI_b_CrashOutpSts input boolean; SI_b_FLDoorButton input boolean; SI_b_FRDoorButton input boolean; SI_b_RLDoorButton input boolean; SI_b_RRDoorButton input boolean; SO_b_FRDoorInnerSwtSts output boolean; SO_b_RLDoorInnerSwtSts output boolean; SO_b_RRDoorInnerSwtSts output boolean

== stateflow chart RELOrigin/REL/DrvDoorUnlockAutoOpen ==
  state InitialSet (E2value) [function]
    (default) -> (junction 74)
    (junction 74) -> (junction 76) [order 1] : [SI_e_BdcDrvrDoorLockSetSts==1]
        | {SO_b_BdcDrvrDoorLockSetSts=1;}
    (junction 74) -> (junction 78) [order 2]
    (junction 78) -> (junction 80) : {SO_b_BdcDrvrDoorLockSetSts=0;}
  state Initial
    en:
    InitialSet(SI_e_BdcDrvrDoorLockSetSts);
  state CFG_SETTING
    CFG_SETTING -> (junction 56)
    (junction 56) -> (junction 58) [order 1] : [SI_e_CdcDrvrDoorLockSet==1]
        | {SO_b_BdcDrvrDoorLockSetSts=1;
        | SO_b_E2BdcDrvrDoorLockSetSts=1;}
    (junction 56) -> (junction 60) [order 2]
    (junction 60) -> (junction 62) : {SO_b_BdcDrvrDoorLockSetSts=0;
        | SO_b_E2BdcDrvrDoorLockSetSts=0;}
  (default) -> Initial
  Initial -> CFG_SETTING : [after(100,tick)]
  data: E2value function_input double; SO_b_BdcDrvrDoorLockSetSts output boolean; SI_e_BdcDrvrDoorLockSetSts input uint8; SI_e_CdcDrvrDoorLockSet input uint8; SO_b_E2BdcDrvrDoorLockSetSts output boolean

== stateflow chart RELOrigin/REL/InnerButtonDrv ==
  state Initial
    en:
    SO_b_DoublePressSucc=0;
  state ONCE
  state TWICE
    en:
    SO_b_DoublePressSucc=1;
  (default) -> Initial
  Initial -> ONCE : [hasChangedTo(SI_b_FLDoorButton,1)]
  ONCE -> TWICE [order 1] : [before(SI_e_DoublePressTime,tick)&&...
      | hasChangedTo(SI_b_FLDoorButton,1)]
  ONCE -> Initial [order 2] : [after(SI_e_DoublePressTime,tick)]
  TWICE -> Initial : [after(3,tick)]
  data: SO_b_DoublePressSucc output boolean; SI_b_FLDoorButton input boolean; SI_e_DoublePressTime input uint8

== stateflow chart RELOrigin/REL/PassInnDoorRat ==
  state Initial
    en:
    SO_b_FRDoorRatReleaseReq=0;
    SO_b_RLDoorRatReleaseReq=0;
    SO_b_RRDoorRatReleaseReq=0;
    SO_DLKUnlockReq=0;
  state TRIGGER
    state RELEASE
      (default) -> (junction 88)
      (junction 88) -> (junction 91) [order 1] : [SI_e_FRDoorRatSts!=3]
      (junction 88) -> (junction 90) [order 2]
      (junction 91) -> (junction 94) : {SO_b_FRDoorRatReleaseReq=1;}
      (junction 94) -> (junction 90)
      (junction 90) -> (junction 97)
      (junction 97) -> (junction 100) [order 1] : [SI_e_RLDoorRatSts!=3]
      (junction 97) -> (junction 103) [order 2]
      (junction 100) -> (junction 99) : {SO_b_RLDoorRatReleaseReq=1;}
      (junction 99) -> (junction 103)
      (junction 103) -> (junction 112)
      (junction 112) -> (junction 109) [order 1] : [SI_e_RRDoorRatSts!=3]
      (junction 112) -> (junction 108) [order 2]
      (junction 109) -> (junction 105) : {SO_b_RRDoorRatReleaseReq=1;}
      (junction 105) -> (junction 108)
    state DOOR_LOCK
      state REQ_UNLOCK
        en:
        SO_DLKUnlockReq=1;
      state SUCESS_UNLOCK
      state FAIL_UNLOCK
      (default) -> REQ_UNLOCK
      REQ_UNLOCK -> SUCESS_UNLOCK [order 1] : [SI_e_DoorLockSts==1]
      REQ_UNLOCK -> FAIL_UNLOCK [order 2] : [after(100,tick)&&...
          | SI_e_DoorLockSts==0]
    state DOOR_UNLOCK
    (default) -> DOOR_LOCK [order 1] : [SI_e_DoorLockSts==0]
    DOOR_LOCK -> RELEASE : [SI_e_DoorLockSts==1&&...
        | (SI_e_FRDoorRatSts!=3||...
        | SI_e_RLDoorRatSts!=3||...
        | SI_e_RRDoorRatSts!=3)]
    DOOR_UNLOCK -> RELEASE : [SI_e_DoorLockSts==1&&...
        | (SI_e_FRDoorRatSts!=3||...
        | SI_e_RLDoorRatSts!=3||...
        | SI_e_RRDoorRatSts!=3)]
    (default) -> DOOR_UNLOCK [order 2]
  (default) -> Initial
  Initial -> TRIGGER : [((SI_e_EspVehSpd<=0&&SI_b_EspVehSpdVld==0)||...
      | SI_e_VcuGearPosn==1)&&...
      | hasChangedTo(SI_b_DoublePressSucc,1)]
  TRIGGER -> Initial [order 1] : [hasChangedFrom(SI_e_VcuGearPosn,1)||...
      | (SI_e_EspVehSpd>=5&&SI_b_EspVehSpdVld==0)||...
      | (after(105,tick)&&SI_e_DoorLockSts==0)]
  TRIGGER -> Initial [order 2] : [SI_e_DoorLockSts==1&&...
      | SI_e_FRDoorRatSts==3&&...
      | SI_e_RLDoorRatSts==3&&...
      | SI_e_RRDoorRatSts==3]
  RELEASE -> (junction 82) : [after(5,tick)]
  (junction 82) -> Initial
  data: SI_e_DoorLockSts input uint8; SI_e_EspVehSpd input uint8; SI_b_EspVehSpdVld input boolean; SI_b_DoublePressSucc input boolean; SI_e_FRDoorRatSts input uint8; SO_DLKUnlockReq output boolean; SO_b_FRDoorRatReleaseReq output boolean; SI_e_VcuGearPosn input uint8; SI_e_RRDoorRatSts input uint8; SI_e_RLDoorRatSts input uint8; SO_b_RLDoorRatReleaseReq output boolean; SO_b_RRDoorRatReleaseReq output boolean

== stateflow chart RELOrigin/REL/InnerButtonPass ==
  state MAIN_JUDGE [group]
    state FR_BUTTON [parallel]
      settings: executionOrder=1
      state Initial
        en:
        SL_b_FRDBLPressSucc=0;
      state ONCE
      state TWICE
        en:
        SL_b_FRDBLPressSucc=1;
      (default) -> MAIN_JUDGE.FR_BUTTON.Initial
      MAIN_JUDGE.FR_BUTTON.Initial -> MAIN_JUDGE.FR_BUTTON.ONCE : [hasChangedTo(SL_b_FRDoorInnerSwtSts,1)]
      MAIN_JUDGE.FR_BUTTON.ONCE -> MAIN_JUDGE.FR_BUTTON.TWICE [order 1] : [before(SI_e_DoublePressTime,tick)&&...
          | hasChangedTo(SL_b_FRDoorInnerSwtSts,1)]
      MAIN_JUDGE.FR_BUTTON.ONCE -> MAIN_JUDGE.FR_BUTTON.Initial [order 2] : [after(SI_e_DoublePressTime,tick)]
      MAIN_JUDGE.FR_BUTTON.TWICE -> MAIN_JUDGE.FR_BUTTON.Initial : [after(3,tick)]
    state RL_BUTTON [parallel]
      settings: executionOrder=2
      state Initial
        en:
        SL_b_RLDBLPressSucc=0;
      state ONCE
      state TWICE
        en:
        SL_b_RLDBLPressSucc=1;
      (default) -> MAIN_JUDGE.RL_BUTTON.Initial
      MAIN_JUDGE.RL_BUTTON.Initial -> MAIN_JUDGE.RL_BUTTON.ONCE : [hasChangedTo(SL_b_RLDoorInnerSwtSts,1)&&...
          | SI_b_LRChildLckSt==0]
      MAIN_JUDGE.RL_BUTTON.ONCE -> MAIN_JUDGE.RL_BUTTON.Initial [order 2] : [after(SI_e_DoublePressTime,tick)||...
          | SI_b_LRChildLckSt==0]
      MAIN_JUDGE.RL_BUTTON.ONCE -> MAIN_JUDGE.RL_BUTTON.TWICE [order 1] : [before(SI_e_DoublePressTime,tick)&&...
          | SI_b_LRChildLckSt==0&&...
          | hasChangedTo(SL_b_RLDoorInnerSwtSts,1)]
      MAIN_JUDGE.RL_BUTTON.TWICE -> MAIN_JUDGE.RL_BUTTON.Initial : [after(3,tick)]
    state RR_BUTTON [parallel]
      settings: executionOrder=3
      state Initial
        en:
        SL_b_RRDBLPressSucc=0;
      state ONCE
      state TWICE
        en:
        SL_b_RRDBLPressSucc=1;
      (default) -> MAIN_JUDGE.RR_BUTTON.Initial
      MAIN_JUDGE.RR_BUTTON.Initial -> MAIN_JUDGE.RR_BUTTON.ONCE : [hasChangedTo(SL_b_RRDoorInnerSwtSts,1)&&...
          | SI_b_RRChildLckSt==0]
      MAIN_JUDGE.RR_BUTTON.ONCE -> MAIN_JUDGE.RR_BUTTON.Initial [order 2] : [after(SI_e_DoublePressTime,tick)||...
          | SI_b_RRChildLckSt!=0]
      MAIN_JUDGE.RR_BUTTON.ONCE -> MAIN_JUDGE.RR_BUTTON.TWICE [order 1] : [before(SI_e_DoublePressTime,tick)&&...
          | SI_b_RRChildLckSt==0&&...
          | hasChangedTo(SL_b_RRDoorInnerSwtSts,1)]
      MAIN_JUDGE.RR_BUTTON.TWICE -> MAIN_JUDGE.RR_BUTTON.Initial : [after(3,tick)]
  state OUTPUT_HANDLE [group]
    state OUTPUT [parallel]
      settings: executionOrder=1
      state IDLE
        en:
        SO_b_DoublePressSucc=0;
      state SEND_OUT
        en:
        SO_b_DoublePressSucc=1;
      (default) -> IDLE
      IDLE -> SEND_OUT : [SL_b_FRDBLPressSucc||...
          | SL_b_RLDBLPressSucc||...
          | SL_b_RRDBLPressSucc]
      SEND_OUT -> IDLE : [!SL_b_FRDBLPressSucc&&...
          | !SL_b_RLDBLPressSucc&&...
          | !SL_b_RRDBLPressSucc]
  data: SO_b_DoublePressSucc output boolean; SL_b_FRDoorInnerSwtSts input boolean; SI_e_DoublePressTime input uint8; SI_b_LRChildLckSt input boolean; SI_b_RRChildLckSt input boolean; SL_b_RLDoorInnerSwtSts input boolean; SL_b_RRDoorInnerSwtSts input boolean; SL_b_FRDBLPressSucc local boolean; SL_b_RRDBLPressSucc local boolean; SL_b_RLDBLPressSucc local boolean

== matlab function RELOrigin/REL/FLDoorRatSts ==
  data: SI_b_DoorAjarSwt input boolean; SO_e_DoorRatSts output uint8; SI_b_DoorSlideAjar input boolean
function SO_e_DoorRatSts = fcn(SI_b_DoorAjarSwt, SI_b_DoorSlideAjar)

aVarTruthTableCondition_1 = false;
aVarTruthTableCondition_2 = false;


% Example condition 1

aVarTruthTableCondition_1 = logical(SI_b_DoorAjarSwt==false);

% Example condition 2

aVarTruthTableCondition_2 = logical(SI_b_DoorSlideAjar==false);

if (~aVarTruthTableCondition_1 && ~aVarTruthTableCondition_2)
    aFcnTruthTableAction_2();
elseif (~aVarTruthTableCondition_1 && aVarTruthTableCondition_2)
    aFcnTruthTableAction_3();
elseif (aVarTruthTableCondition_1 && aVarTruthTableCondition_2)
    aFcnTruthTableAction_4();
else % Default
    aFcnTruthTableAction_1();
end

function aFcnTruthTableAction_1()

% Invalid

SO_e_DoorRatSts=0;

function aFcnTruthTableAction_2()

% All Lock

SO_e_DoorRatSts=1;

function aFcnTruthTableAction_3()

% Half Lock

SO_e_DoorRatSts=2;

function aFcnTruthTableAction_4()

% All Unlock

SO_e_DoorRatSts=3;

== matlab function RELOrigin/REL/FRDoorRatSts ==
  data: SI_b_DoorAjarSwt input boolean; SO_e_DoorRatSts output uint8; SI_b_DoorSlideAjar input boolean
function SO_e_DoorRatSts = fcn(SI_b_DoorAjarSwt, SI_b_DoorSlideAjar)

aVarTruthTableCondition_1 = false;
aVarTruthTableCondition_2 = false;


% Example condition 1

aVarTruthTableCondition_1 = logical(SI_b_DoorAjarSwt==false);

% Example condition 2

aVarTruthTableCondition_2 = logical(SI_b_DoorSlideAjar==false);

if (~aVarTruthTableCondition_1 && ~aVarTruthTableCondition_2)
    aFcnTruthTableAction_2();
elseif (~aVarTruthTableCondition_1 && aVarTruthTableCondition_2)
    aFcnTruthTableAction_3();
elseif (aVarTruthTableCondition_1 && aVarTruthTableCondition_2)
    aFcnTruthTableAction_4();
else % Default
    aFcnTruthTableAction_1();
end

function aFcnTruthTableAction_1()

% Invalid

SO_e_DoorRatSts=0;

function aFcnTruthTableAction_2()

% All Lock

SO_e_DoorRatSts=1;

function aFcnTruthTableAction_3()

% Half Lock

SO_e_DoorRatSts=2;

function aFcnTruthTableAction_4()

% All Unlock

SO_e_DoorRatSts=3;

== matlab function RELOrigin/REL/RLDoorRatSts ==
  data: SI_b_DoorAjarSwt input boolean; SO_e_DoorRatSts output uint8; SI_b_DoorSlideAjar input boolean
function SO_e_DoorRatSts = fcn(SI_b_DoorAjarSwt, SI_b_DoorSlideAjar)

aVarTruthTableCondition_1 = false;
aVarTruthTableCondition_2 = false;


% Example condition 1

aVarTruthTableCondition_1 = logical(SI_b_DoorAjarSwt==false);

% Example condition 2

aVarTruthTableCondition_2 = logical(SI_b_DoorSlideAjar==false);

if (~aVarTruthTableCondition_1 && ~aVarTruthTableCondition_2)
    aFcnTruthTableAction_2();
elseif (~aVarTruthTableCondition_1 && aVarTruthTableCondition_2)
    aFcnTruthTableAction_3();
elseif (aVarTruthTableCondition_1 && aVarTruthTableCondition_2)
    aFcnTruthTableAction_4();
else % Default
    aFcnTruthTableAction_1();
end

function aFcnTruthTableAction_1()

% Invalid

SO_e_DoorRatSts=0;

function aFcnTruthTableAction_2()

% All Lock

SO_e_DoorRatSts=1;

function aFcnTruthTableAction_3()

% Half Lock

SO_e_DoorRatSts=2;

function aFcnTruthTableAction_4()

% All Unlock

SO_e_DoorRatSts=3;

== matlab function RELOrigin/REL/RRDoorRatSts ==
  data: SI_b_DoorAjarSwt input boolean; SO_e_DoorRatSts output uint8; SI_b_DoorSlideAjar input boolean
function SO_e_DoorRatSts = fcn(SI_b_DoorAjarSwt, SI_b_DoorSlideAjar)

aVarTruthTableCondition_1 = false;
aVarTruthTableCondition_2 = false;


% Example condition 1

aVarTruthTableCondition_1 = logical(SI_b_DoorAjarSwt==false);

% Example condition 2

aVarTruthTableCondition_2 = logical(SI_b_DoorSlideAjar==false);

if (~aVarTruthTableCondition_1 && ~aVarTruthTableCondition_2)
    aFcnTruthTableAction_2();
elseif (~aVarTruthTableCondition_1 && aVarTruthTableCondition_2)
    aFcnTruthTableAction_3();
elseif (aVarTruthTableCondition_1 && aVarTruthTableCondition_2)
    aFcnTruthTableAction_4();
else % Default
    aFcnTruthTableAction_1();
end

function aFcnTruthTableAction_1()

% Invalid

SO_e_DoorRatSts=0;

function aFcnTruthTableAction_2()

% All Lock

SO_e_DoorRatSts=1;

function aFcnTruthTableAction_3()

% Half Lock

SO_e_DoorRatSts=2;

function aFcnTruthTableAction_4()

% All Unlock

SO_e_DoorRatSts=3;

== stateflow chart RELOrigin/REL/Request_DLK_Unlock ==
  state REQ_SENT
    REQ_SENT -> (junction 56) [order 1]
    (junction 56) -> (junction 58) [order 1] : [SL_DLKDrvUnlockReq==1&&...
        | SL_DLKPassUnlockReq==1]
    (junction 56) -> (junction 60) [order 2]
    (junction 58) -> (junction 91) : {SO_e_DLKUnlockReq=3;}
    (junction 60) -> (junction 62) [order 1] : [SL_DLKDrvUnlockReq==1&&...
        | SL_DLKPassUnlockReq!=1]
    (junction 60) -> (junction 84) [order 2]
    (junction 62) -> (junction 93) : {SO_e_DLKUnlockReq=1;}
    (junction 84) -> (junction 83) [order 1] : [SL_DLKDrvUnlockReq!=1&&...
        | SL_DLKPassUnlockReq==1]
    (junction 84) -> (junction 88) [order 2] : {SO_e_DLKUnlockReq=0;}
    (junction 83) -> (junction 95) : {SO_e_DLKUnlockReq=2;}
  state Initial
    en:
    SO_e_DLKUnlockReq=0;
  (default) -> Initial
  Initial -> REQ_SENT : [hasChangedTo(SL_DLKDrvUnlockReq,1)||...
      | hasChangedTo(SL_DLKPassUnlockReq,1)]
  REQ_SENT -> Initial [order 1] : [SL_DLKDrvUnlockReq==0&&...
      | SL_DLKPassUnlockReq==0]
  data: SO_e_DLKUnlockReq output uint8; SL_DLKDrvUnlockReq input boolean; SL_DLKPassUnlockReq input boolean

== stateflow chart RELOrigin/REL/FLElecDoorRat ==
  state Initial
    en:
    SO_b_DoorRatRelaseReq=0;
  state RELEASE
    en:
    SO_b_DoorRatRelaseReq=1;
  (default) -> Initial
  Initial -> RELEASE : [!SI_b_OFF&&...
      | SI_e_DoorLockSts==1&&...
      | SI_e_DoorRatSts!=3&&...
      | ((SI_e_EspVehSpd<=0&&SI_b_EspVehSpdVld==0)||...
      | SI_e_VcuGearPosn==1)&&...
      | ((SI_b_BdcDrvrDoorLockSetSts==1&&SI_b_BDCDrvrDoorOpenReq)||...
      | (SI_e_BDCDoorHndSts==1&&hasChangedTo(SI_b_DoorHandleSW,1))||...
      | (SI_e_VcuGearPosn==1&&hasChangedTo(SI_e_BTDoorOpenReq,1))||...
      | (SI_e_VcuGearPosn==1&&hasChangedTo(SI_e_BTDoorOpenReq,9)))]
  RELEASE -> Initial : [after(5,tick)]
  data: SI_b_OFF input boolean; SO_b_DoorRatRelaseReq output boolean; SI_e_DoorLockSts input uint8; SI_e_EspVehSpd input uint8; SI_b_EspVehSpdVld input boolean; SI_e_DoorRatSts input uint8; SI_e_VcuGearPosn input uint8; SI_b_BdcDrvrDoorLockSetSts input boolean; SI_b_BDCDrvrDoorOpenReq input boolean; SI_e_BDCDoorHndSts input uint8; SI_b_DoorHandleSW input boolean; SI_e_BTDoorOpenReq input uint8

== stateflow chart RELOrigin/REL/FLCenDoorRat ==
  state Initial
    en:
    SO_b_DoorRatRelaseReq=0;
    SO_DLKUnlockReq=0;
  state TRIGGER
    state DOOR_LOCK
      state REQ_UNLOCK
        en:
        SO_DLKUnlockReq=1;
      state SUCESS_UNLOCK
      state FAIL_UNLOCK
      (default) -> REQ_UNLOCK
      REQ_UNLOCK -> SUCESS_UNLOCK [order 1] : [SI_e_DoorLockSts==1]
      REQ_UNLOCK -> FAIL_UNLOCK [order 2] : [after(100,tick)&&...
          | SI_e_DoorLockSts==0]
    state RELEASE
      en:
      SO_b_DoorRatRelaseReq=1;
    state DOOR_UNLOCK
    (default) -> DOOR_LOCK [order 1] : [SI_e_DoorLockSts==0]
    DOOR_LOCK -> RELEASE : [SI_e_DoorLockSts==1&&...
        | SI_e_DoorRatSts!=3]
    DOOR_UNLOCK -> RELEASE : [SI_e_DoorLockSts==1&&...
        | SI_e_DoorRatSts!=3]
    (default) -> DOOR_UNLOCK [order 2]
  (default) -> Initial
  Initial -> TRIGGER : [!SI_b_OFF&&...
      | SI_e_DoorRatSts!=3&&...
      | ((SI_e_EspVehSpd<=0&&SI_b_EspVehSpdVld==0)||...
      | SI_e_VcuGearPosn==1)&&...
      | (hasChangedTo(SI_b_CdcDoorButtonSts,1)||...
      | hasChangedTo(SI_b_Cdc4DoorOpenButtonSts,1))]
  TRIGGER -> Initial : [hasChangedFrom(SI_e_VcuGearPosn,1)||...
      | (SI_e_EspVehSpd>=5&&SI_b_EspVehSpdVld==0)||...
      | (after(105,tick)&&SI_e_DoorLockSts==0)]
  RELEASE -> (junction 82) : [after(5,tick)]
  (junction 82) -> Initial
  data: SI_b_OFF input boolean; SO_b_DoorRatRelaseReq output boolean; SI_e_DoorLockSts input uint8; SI_e_EspVehSpd input uint8; SI_b_EspVehSpdVld input boolean; SI_e_DoorRatSts input uint8; SO_DLKUnlockReq output boolean; SI_e_VcuGearPosn input uint8; SI_b_CdcDoorButtonSts input boolean; SI_b_Cdc4DoorOpenButtonSts input boolean

== stateflow chart RELOrigin/REL/FRElecDoorRat ==
  state Initial
    en:
    SO_b_DoorRatRelaseReq=0;
  state RELEASE
    en:
    SO_b_DoorRatRelaseReq=1;
  (default) -> Initial
  Initial -> RELEASE : [!SI_b_OFF&&...
      | SI_e_DoorLockSts==1&&...
      | SI_e_DoorRatSts!=3&&...
      | ((SI_e_EspVehSpd<=0&&SI_b_EspVehSpdVld==0)||...
      | SI_e_VcuGearPosn==1)&&...
      | ((SI_e_BDCDoorHndSts==1&&hasChangedTo(SI_b_DoorHandleSW,1))||...
      | (SI_e_VcuGearPosn==1&&hasChangedTo(SI_e_BTDoorOpenReq,3))||...
      | (SI_e_VcuGearPosn==1&&hasChangedTo(SI_e_BTDoorOpenReq,9)))]
  RELEASE -> Initial : [after(5,tick)]
  data: SI_b_OFF input boolean; SO_b_DoorRatRelaseReq output boolean; SI_e_DoorLockSts input uint8; SI_e_EspVehSpd input uint8; SI_b_EspVehSpdVld input boolean; SI_e_DoorRatSts input uint8; SI_e_VcuGearPosn input uint8; SI_e_BDCDoorHndSts input uint8; SI_b_DoorHandleSW input boolean; SI_e_BTDoorOpenReq input uint8

== stateflow chart RELOrigin/REL/FLInnDoorRat ==
  state Initial
    en:
    SO_b_DoorRatRelaseReq=0;
    SO_DLKUnlockReq=0;
  state TRIGGER
    state DOOR_LOCK
      state REQ_UNLOCK
        en:
        SO_DLKUnlockReq=1;
      state SUCESS_UNLOCK
      state FAIL_UNLOCK
      (default) -> REQ_UNLOCK
      REQ_UNLOCK -> SUCESS_UNLOCK [order 1] : [SI_e_DoorLockSts==1]
      REQ_UNLOCK -> FAIL_UNLOCK [order 2] : [after(100,tick)&&...
          | SI_e_DoorLockSts==0]
    state RELEASE
      en:
      SO_b_DoorRatRelaseReq=1;
    state DOOR_UNLOCK
    (default) -> DOOR_LOCK [order 1] : [SI_e_DoorLockSts==0]
    DOOR_LOCK -> RELEASE : [SI_e_DoorLockSts==1&&...
        | SI_e_DoorRatSts!=3]
    DOOR_UNLOCK -> RELEASE : [SI_e_DoorLockSts==1&&...
        | SI_e_DoorRatSts!=3]
    (default) -> DOOR_UNLOCK [order 2]
  (default) -> Initial
  Initial -> TRIGGER : [((SI_e_EspVehSpd<=0&&SI_b_EspVehSpdVld==0)||...
      | SI_e_VcuGearPosn==1)&&...
      | hasChangedTo(SI_b_DoublePressSucc,1)]
  TRIGGER -> Initial [order 1] : [hasChangedFrom(SI_e_VcuGearPosn,1)||...
      | (SI_e_EspVehSpd>=5&&SI_b_EspVehSpdVld==0)||...
      | (after(105,tick)&&SI_e_DoorLockSts==0)]
  TRIGGER -> Initial [order 2] : [SI_e_DoorLockSts==1&&...
      | SI_e_DoorRatSts==3]
  RELEASE -> (junction 82) : [after(5,tick)]
  (junction 82) -> Initial
  data: SO_b_DoorRatRelaseReq output boolean; SI_e_DoorLockSts input uint8; SI_e_EspVehSpd input uint8; SI_b_EspVehSpdVld input boolean; SI_b_DoublePressSucc input boolean; SI_e_DoorRatSts input uint8; SO_DLKUnlockReq output boolean; SI_e_VcuGearPosn input uint8
